simulink model "DCmotorPractice"  (R2020b)
settings: Solver=VariableStepAuto  StartTime=0.0  StopTime=10.0  RelTol=1e-3
values from neighbouring files (symbols this model uses):
  K = 2    [Test2_1.m]
undefined symbols (not defined in the file or in its folder): D, J_L, J_M, K_E, K_T, L
settings Model: Creator=yuto  LastModifiedBy=yuto

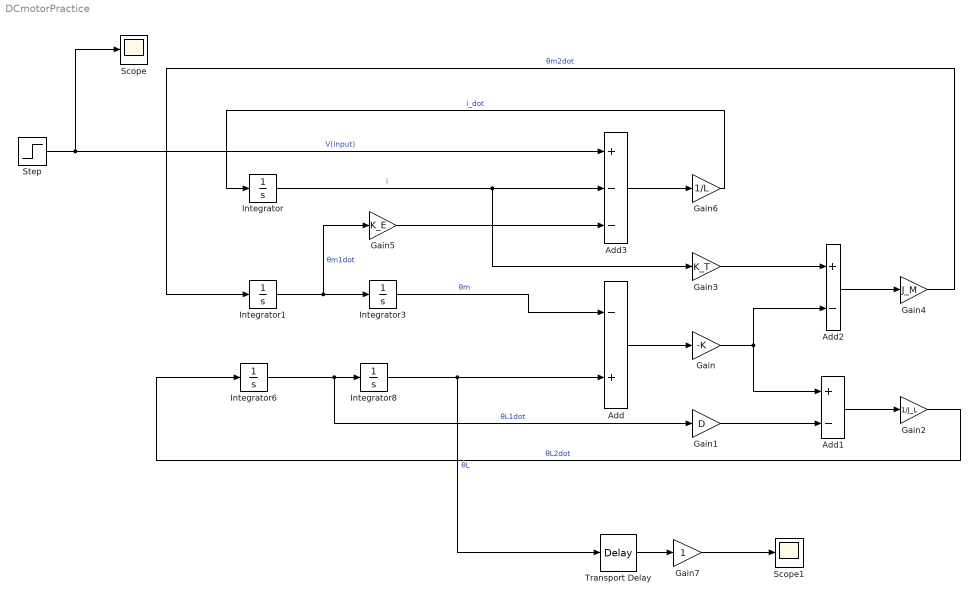
== system DCmotorPractice ==
  Add : Sum  Inputs=-+
  Add1 : Sum  Inputs=+-
  Add2 : Sum  Inputs=+-
  Add3 : Sum  Inputs=+--
  Gain : Gain  Gain=-K
  Gain1 : Gain  Gain=D
  Gain2 : Gain  Gain=1/J_L
  Gain3 : Gain  Gain=K_T
  Gain4 : Gain  Gain=J_M
  Gain5 : Gain  Gain=K_E
  Gain6 : Gain  Gain=1/L
  Gain7 : Gain
  Integrator{,1,3,6,8} (5 alike) : Integrator
  Scope : Scope
  Scope1 : Scope
  Step : Step  SampleTime=0
  Transport Delay : TransportDelay
  wires:
  Integrator/1 -> Gain3/1, Add3/2  "i"
  Integrator1/1 -> Gain5/1, Integrator3/1  "θm1dot"
  Integrator3/1 -> Add/1  "θm"
  Integrator8/1 -> Transport Delay/1, Add/2  "θL"
  Integrator6/1 -> Gain1/1, Integrator8/1  "θL1dot"
  Add/1 -> Gain/1
  Gain1/1 -> Add1/2
  Add1/1 -> Gain2/1
  Gain/1 -> Add1/1, Add2/2
  Gain2/1 -> Integrator6/1  "θL2dot"
  Gain3/1 -> Add2/1
  Add2/1 -> Gain4/1
  Gain4/1 -> Integrator1/1  "θm2dot"
  Step/1 -> Scope/1, Add3/1  "V(input)"
  Gain5/1 -> Add3/3
  Add3/1 -> Gain6/1
  Gain6/1 -> Integrator/1  "i_dot"
  Transport Delay/1 -> Gain7/1
  Gain7/1 -> Scope1/1
